simulink model "slexEntityTransportDelay"  (R2024a)
settings: Solver=VariableStepAuto  StartTime=0.0  StopTime=900  RelTol=1e-3
PostLoadFcn:
  | Simulink.defineIntEnumType('OperationMode', {'Idle', 'OnDemand', 'Max'}, [0; 1; 2]);
undefined symbols (not defined in the file): m, n
Description:
  | <include>VariableSpeedConveyorBeltExample.m</include>
settings Model: PacingRate=1000  Creator=The MathWorks, Inc.  LastModifiedBy=uditpant
settings SolverCC: AlgebraicLoopSolver=TrustRegion
settings DebuggingCC: UnconnectedInputMsg=warning  UnconnectedOutputMsg=warning  UnconnectedLineMsg=warning  StrictBusMsg=ErrorOnBusTreatedAsVector  SymbolicDimsDataTypeCodeGenerationDiagnostic=none
settings ModelReferenceCC: EnableRefExpFcnMdlSchedulingChecks=on
settings RTWCC: GPUComputeCapability=3.5

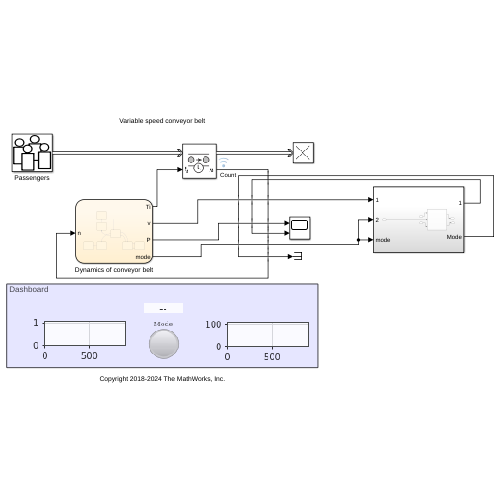
[thumbnail: Simulink's stored preview of the top-level diagram]
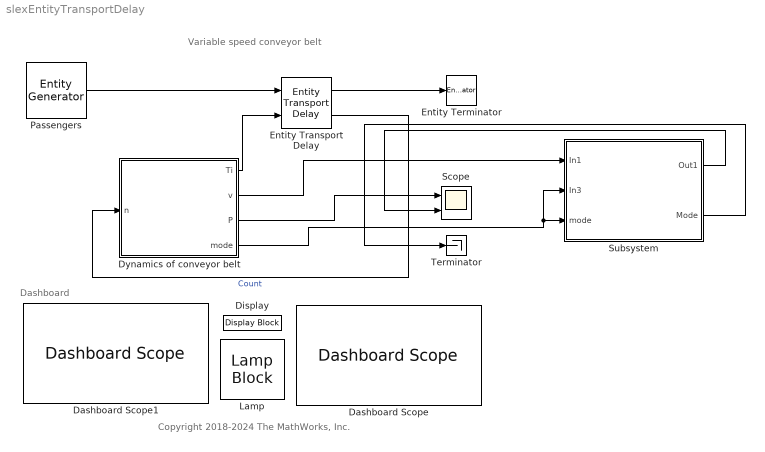
== system slexEntityTransportDelay ==
  note: Dashboard
  note: Copyright 2018-2024 The MathWorks, Inc.
  note: Variable speed conveyor belt
  Dashboard Scope : DashboardScope  Ymin=0  Ymax=110
  Dashboard Scope1 : DashboardScope  Ymin=0  Ymax=1.1000000000000001
  Display : DisplayBlock  LabelPosition=Hide  Transparency=1
  Dynamics of conveyor belt : Stateflow chart  TreatAsAtomicUnit=on
  Entity Transport Delay : EntityTransportDelay  InputPortMessageModes=m,n  OutputPortMessageModes=m,n  ShowNumberEntitiesInBlock=on
  Entity Terminator : EntityTerminator  InputPortMessageModes=m
  Lamp : LampBlock
  Passengers : EntityGenerator  OutputPortMessageModes=m  TimeSource=MATLAB action  Period=0.1  IntergenerationTimeAction=|  GenerateEntityAtSimulationStart=off  EntityType=Structured  EntityTypeName=Entity
      | persistent rngInit;
      | if isempty(rngInit)
      |     seed = 12345;
      |     rng(seed);
      |     rngInit = true;
      | end
      | 
      | % Pattern: Exponential distribution
      | persistent time;
      | if isempty(time)
      |     time = 0;
      | end
      | if time < 180
      |     lambda = 2;
      | elseif time < 240
      |     lambda = .5;
      | elseif time < 300
      |     lambda = .1;
      | else
      |     time = 0;
      |     lambda = 2;
      | end
      | % Use inverse transform sampling to
      | % generate dt according to the exponential
      | % distribution
      | dt = -1/lambda * log(1 - rand());
      | time = time + dt;
      mask Display: image('$imagefile'); % Use "Edit Image" on toolstrip to change.
  Scope : Scope  NumInputPorts=2
  Subsystem : Subsystem
  Terminator : Terminator
  wires:
  Entity Transport Delay/1 -> Entity Terminator/1
  Dynamics of conveyor belt/1(Ti) -> Entity Transport Delay/2
  Entity Transport Delay/2 -> Dynamics of conveyor belt/1(n)  "Count"
  Passengers/1 -> Entity Transport Delay/1
  Dynamics of conveyor belt/2(v) -> Subsystem/1(In1)
  Dynamics of conveyor belt/4(mode) -> Subsystem/3(mode), Subsystem/2(In3)
  Subsystem/1(Out1) -> Scope/2
  Subsystem/2(Mode) -> Terminator/1
  Dynamics of conveyor belt/3(P) -> Scope/1

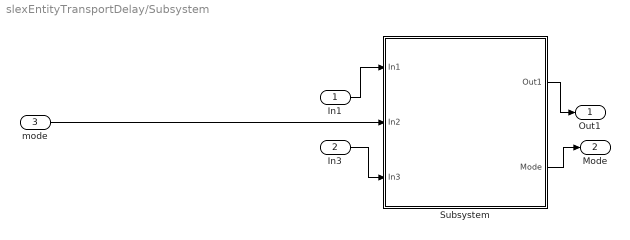
== system slexEntityTransportDelay/Subsystem ==
  In1 : Inport
  In3 : Inport  Port=2
  mode : Inport  Port=3
  Subsystem : Subsystem
  Out1 : Outport
  Mode : Outport  Port=2
  wires:
  In1/1 -> Subsystem/1(In1)
  mode/1 -> Subsystem/2(In2)
  In3/1 -> Subsystem/3(In3)
  Subsystem/1(Out1) -> Out1/1
  Subsystem/2(Mode) -> Mode/1

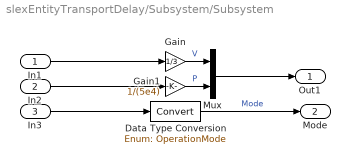
== system slexEntityTransportDelay/Subsystem/Subsystem ==
  In1 : Inport
  In2 : Inport  Port=2
  In3 : Inport  Port=3
  Data Type Conversion : DataTypeConversion  OutDataTypeStr=Enum: OperationMode  SaturateOnIntegerOverflow=off  RndMeth=Floor
  Gain : Gain  Gain=1/3
  Gain1 : Gain  Gain=1/(5e4)
  Mux : Mux  Inputs=2
  Out1 : Outport
  Mode : Outport  Port=2
  wires:
  Gain1/1 -> Mux/2  "P"
  In3/1 -> Data Type Conversion/1
  Mux/1 -> Out1/1
  Gain/1 -> Mux/1  "V"
  In1/1 -> Gain/1
  In2/1 -> Gain1/1
  Data Type Conversion/1 -> Mode/1  "Mode"

== stateflow chart slexEntityTransportDelay/Dynamics of conveyor belt ==
  state OnDemand1
    % keep speed
    Ti=L/V;
    v=V;
    P=(mu*n+fBelt)*v;
    mode=1;
  state OffDemand1
    % keep speed
    Ti=L/V;
    v=V;
    P=(mu*n+fBelt)*v;
    mode=1;
  state Idle
    % no load
    Ti=100;
    v=1/Ti*L;
    P=(mu*n+fBelt)*v;
    mode=0;
  state Max2
    % keep power
    v=maxPower/(mu*n+fBelt);
    Ti = L/v;
    P=(mu*n+fBelt)*v;
    mode=2;
  state Max1
    % keep power
    v=maxPower/(mu*n+fBelt);
    Ti = L/v;
    P=(mu*n+fBelt)*v;
    mode=2;
  state OnDemand
    % keep speed
    Ti=L/V;
    v=V;
    P=(mu*n+fBelt)*v;
    mode=1;
  state Max
    % keep power
    v=maxPower/(mu*n+fBelt);
    Ti = L/v;
    P=(mu*n+fBelt)*v;
    mode=2;
  (default) -> Idle [order 1] : {
      | % initialize local parameters
      | aveMass = 75;
      | mu = 0.5*10*aveMass; % *mu*g*aveMass, [N]
      | maxPower = 5e4; % maximum power, [W]
      | V = 3; % normal mode velocity, [m/s]
      | L = 50; % length of belt, [L]
      | fBelt = 1e4; % friction of zero load, [N]
      | }
  OffDemand1 -> OnDemand1
  (default) -> OffDemand1 [order 2]
  Idle -> OffDemand1 [order 3]
  Idle -> OnDemand [order 1] : [n*aveMass >= 10]
  Idle -> Max1 [order 2]
  OnDemand -> Idle [order 1] : [n*aveMass < 10]
  OnDemand -> Max [order 2] : [(maxPower/V-fBelt)/mu  <= n]
  Max1 -> Max2
  Max -> OnDemand : [(maxPower/V-fBelt)/mu > n]
  data: Ti output; n input; mu local double =50; maxPower local double =5e4; V local double =3; L local double =50; fBelt local double =1e4; v output; P output; mode output int8; aveMass local
